simulink model "Model_2"  (R2020b)
settings: Solver=VariableStepAuto  StartTime=0.0  StopTime=10.0  RelTol=1e-3
undefined symbols (not defined in the file): DiscIntNeverNeededParam
libraries: simulink x1
settings Model: Creator=samar  LastModifiedBy=samar

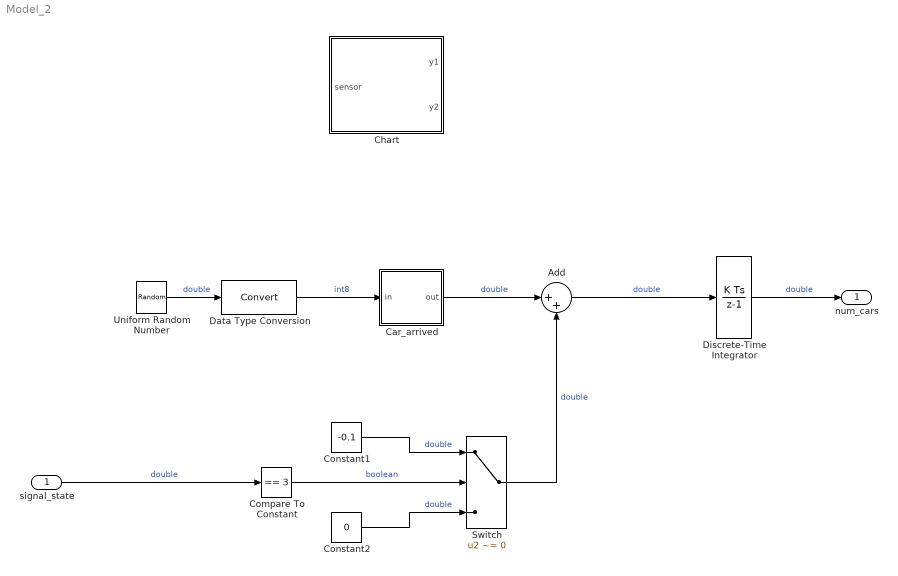
== system Model_2 ==
  signal_state : Inport
  Add : Sum  Inputs=|++
  Car_arrived : Stateflow chart  TreatAsAtomicUnit=on
  Chart : Stateflow chart  TreatAsAtomicUnit=on
  Compare To Constant : simulink/Logic and Bit Operations/Compare To Constant  relop===  const=3  OutDataTypeStr=boolean  ZeroCross=off
  Constant1 : Constant  Value=-0.1
  Constant2 : Constant  Value=0
  Data Type Conversion : DataTypeConversion
  Discrete-Time Integrator : DiscreteIntegrator  SampleTime=-1  LimitOutput=on  LowerSaturationLimit=0  ICPrevOutput=DiscIntNeverNeededParam  ICPrevScaledInput=DiscIntNeverNeededParam
  Switch : Switch  Criteria=u2 ~= 0
  Uniform Random Number : UniformRandomNumber  Minimum=0  Maximum=100  Seed=177836  SampleTime=0
  num_cars : Outport  VectorParamsAs1DForOutWhenUnconnected=off
  wires:
  Uniform Random Number/1 -> Data Type Conversion/1  "double"
  Data Type Conversion/1 -> Car_arrived/1(in)  "int8"
  Car_arrived/1(out) -> Add/1  "double"
  Add/1 -> Discrete-Time Integrator/1  "double"
  Discrete-Time Integrator/1 -> num_cars/1  "double"
  signal_state/1 -> Compare To Constant/1  "double"
  Compare To Constant/1 -> Switch/2  "boolean"
  Constant1/1 -> Switch/1  "double"
  Constant2/1 -> Switch/3  "double"
  Switch/1 -> Add/2  "double"

== stateflow chart Model_2/Chart ==
  state Stop
    y1 = RED;
    y2 = GREEN;
  state Stop_For_Traffic
    y1 = RED;
    y2 = GREEN;
  state Stop_To_Go
    y1 = RED;
    y2 = YELLOW;
  state Go_To_Stop
    y1 = YELLOW;
    y2 = RED;
  state Go
    y1 = GREEN;
    y2 = RED;
  (default) -> Stop
  Stop_For_Traffic -> Stop_To_Go : [sensor]
  Stop -> Stop_For_Traffic : after(20,tick)
  Stop_To_Go -> Go : after(3,tick)
  Go_To_Stop -> Stop : after(3,tick)
  Go -> Go_To_Stop : after(10,tick)
  data: sensor input; y1 output; y2 output; GREEN constant double; RED constant double; YELLOW constant double

== stateflow chart Model_2/Car_arrived ==
  (default) -> (junction 2) : {out = in > 98;}
  data: in input int8; out output double
